simulink model "frontsusp"  (R2018a)
settings: Solver=VariableStepAuto  StartTime=0.0  StopTime=10.0  RelTol=1e-3
settings Model: Creator=Seb  LastModifiedBy=Seb

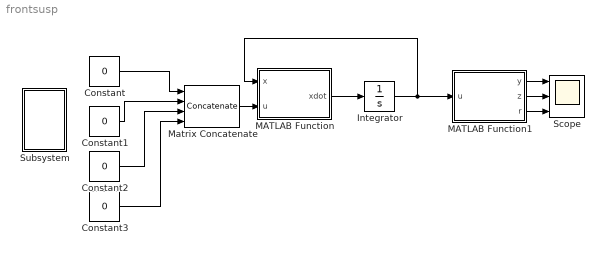
== system frontsusp ==
  Constant{,1..3} (4 alike) : Constant  Value=0
  Integrator : Integrator  InitialCondition=[0 0 0 0 0 0].'
  MATLAB Function : MATLAB Function  TreatAsAtomicUnit=on
  MATLAB Function1 : MATLAB Function  TreatAsAtomicUnit=on
  Matrix Concatenate : Concatenate  NumInputs=4  Mode=Multidimensional array  ConcatenateDimension=2
  Scope : Scope  NumInputPorts=3
  Subsystem : Subsystem
  wires:
  MATLAB Function/1(xdot) -> Integrator/1
  Integrator/1 -> MATLAB Function1/1(u), MATLAB Function/1(x)
  Constant/1 -> Matrix Concatenate/1
  Constant1/1 -> Matrix Concatenate/2
  Constant2/1 -> Matrix Concatenate/3
  Constant3/1 -> Matrix Concatenate/4
  Matrix Concatenate/1 -> MATLAB Function/2(u)
  MATLAB Function1/1(y) -> Scope/1
  MATLAB Function1/2(z) -> Scope/2
  MATLAB Function1/3(r) -> Scope/3

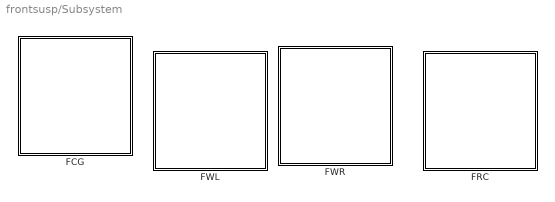
== system frontsusp/Subsystem ==
  FCG : Subsystem  DialogController=hmiCreateDDGDialog  IsWebBlock=on  mask(MWDashboardBlock){webBlockId=e7474ebc-52c4-474b-8036-e4bcff60fafa, webBlockType=continuousknob, ShowInLibBrowser=on, ShowInitialText=on, HMISrcModelName=frontsusp}
      mask prompts: webBlockId "WebBlock Id"; webBlockType "WebBlock Type"; HMISrcModelName "Source Model"
      mask help: SimulinkHMI:dialogs:ContinuousKnobDialogDesc
      mask Help: helpview([docroot '/mapfiles/simulink.map'], 'hmi_knob')
      mask Display:
      | if strcmp(get_param(bdroot(gcb),'BlockDiagramType'), 'library')
      |     image([(matlabroot) '/toolbox/simulink/hmi/icons/ContinuousKnob.png']);
      | end
  FRC : Subsystem  DialogController=hmiCreateDDGDialog  IsWebBlock=on  mask(MWDashboardBlock){webBlockId=dbe03f35-0bda-4943-861c-fa44fdb9e248, webBlockType=continuousknob, ShowInLibBrowser=on, ShowInitialText=on, HMISrcModelName=frontsusp}
      mask prompts: webBlockId "WebBlock Id"; webBlockType "WebBlock Type"; HMISrcModelName "Source Model"
      mask help: SimulinkHMI:dialogs:ContinuousKnobDialogDesc
      mask Help: helpview([docroot '/mapfiles/simulink.map'], 'hmi_knob')
      mask Display:
      | if strcmp(get_param(bdroot(gcb),'BlockDiagramType'), 'library')
      |     image([(matlabroot) '/toolbox/simulink/hmi/icons/ContinuousKnob.png']);
      | end
  FWL : Subsystem  DialogController=hmiCreateDDGDialog  IsWebBlock=on  mask(MWDashboardBlock){webBlockId=6a58f6f3-af90-4d87-bb64-525b631442a4, webBlockType=continuousknob, ShowInLibBrowser=on, ShowInitialText=on, HMISrcModelName=frontsusp}
      mask prompts: webBlockId "WebBlock Id"; webBlockType "WebBlock Type"; HMISrcModelName "Source Model"
      mask help: SimulinkHMI:dialogs:ContinuousKnobDialogDesc
      mask Help: helpview([docroot '/mapfiles/simulink.map'], 'hmi_knob')
      mask Display:
      | if strcmp(get_param(bdroot(gcb),'BlockDiagramType'), 'library')
      |     image([(matlabroot) '/toolbox/simulink/hmi/icons/ContinuousKnob.png']);
      | end
  FWR : Subsystem  DialogController=hmiCreateDDGDialog  IsWebBlock=on  mask(MWDashboardBlock){webBlockId=f9ef0bb1-865b-4ac9-b4c3-7081c3261898, webBlockType=continuousknob, ShowInLibBrowser=on, ShowInitialText=on, HMISrcModelName=frontsusp}
      mask prompts: webBlockId "WebBlock Id"; webBlockType "WebBlock Type"; HMISrcModelName "Source Model"
      mask help: SimulinkHMI:dialogs:ContinuousKnobDialogDesc
      mask Help: helpview([docroot '/mapfiles/simulink.map'], 'hmi_knob')
      mask Display:
      | if strcmp(get_param(bdroot(gcb),'BlockDiagramType'), 'library')
      |     image([(matlabroot) '/toolbox/simulink/hmi/icons/ContinuousKnob.png']);
      | end

== system frontsusp/Subsystem/FCG ==

== system frontsusp/Subsystem/FRC ==

== system frontsusp/Subsystem/FWL ==

== system frontsusp/Subsystem/FWR ==

== matlab function frontsusp/MATLAB Function1 ==
  data: u input; y output; z output; r output
function [y,z,r] = fcn(u)

y = u(1);
z = u(2);
r = u(3);

== matlab function frontsusp/MATLAB Function ==
  data: x input; u input; xdot output
function xdot = fcn(x,u)
%        [k b l h s m I g].';

params = [10000 1000 2 0.3 0.05 150 20 9.81].';
xdot = suspmodel(x,u,params);
